simulink library "vmodel_blocks"  (Simulink 7.3)
settings: Solver=ode45  StartTime=0.0  StopTime=10.0  RelTol=1e-3
settings Model: Creator=labirint  LastModifiedBy=chuh

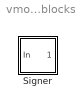
== system vmodel_blocks ==
  Signer : Subsystem  mask(vmodel signer){N=12}
      mask prompts: N "Input width (bit)"
      mask help: Block converts uint32 output into equal signed double

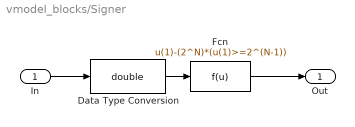
== system vmodel_blocks/Signer ==
  In : Inport  OutDataType=fixdt(1, 16)  OutScaling=2^0
  Data Type Conversion : DataTypeConversion  OutDataTypeMode=double  OutDataType=fixdt(1, 16)  OutScaling=2^0  OutDataTypeStr=double
  Fcn : Fcn  Expr=u(1)-(2^N)*(u(1)>=2^(N-1))
  Out : Outport  OutDataType=fixdt(1, 16)  OutScaling=2^0
  wires:
  Data Type Conversion/1 -> Fcn/1
  Fcn/1 -> Out/1
  In/1 -> Data Type Conversion/1
